simulink model "RoboBoat_CompassGPSlidar"  (R2014a)
settings: Solver=FixedStepDiscrete  StartTime=0.0  StopTime=inf  FixedStep=.1  RelTol=1e-3
undefined symbols (not defined in the file): Com1, Com2, Com3, Com4, DiscIntNeverNeededParam, standard
libraries: xpcseriallib x31, visiontextngfix x25, simulink x19, slrtlib x9, speedgoatlib_IO102 x3, speedgoatlib x2
(part 1 of 4)
settings Model: BufferReuse=off  Creator=wildcat  LastModifiedBy=wildcat
settings SolverCC: EnableConcurrentExecution=on
settings DataIOCC: SignalLoggingSaveFormat=ModelDataLogs
settings OptimizationCC: BlockReduction=off  OptimizeBlockIOStorage=off  BufferReuse=off  GlobalBufferReuse=off  ExpressionFolding=off  LocalBlockOutputs=off
settings DebuggingCC: UnderspecifiedInitializationDetection=Classic  MultiTaskDSMMsg=warning  StateNameClashWarn=warning
settings HardwareCC: ProdIntDivRoundTo=Zero  ProdEndianess=LittleEndian  ProdHWDeviceType=Generic->32-bit x86 compatible
settings RTWCC: SystemTargetFile=slrt.tlc  TemplateMakefile=slrt_default_tmf  Description=Simulink Real-Time  ProcessScript=slrt_make_rtw_hook  RTWCompilerOptimization=On
settings SimulinkRealTimeCC: GeneratePreprocessorConditionals=Disable all  EnableShiftOperators=on

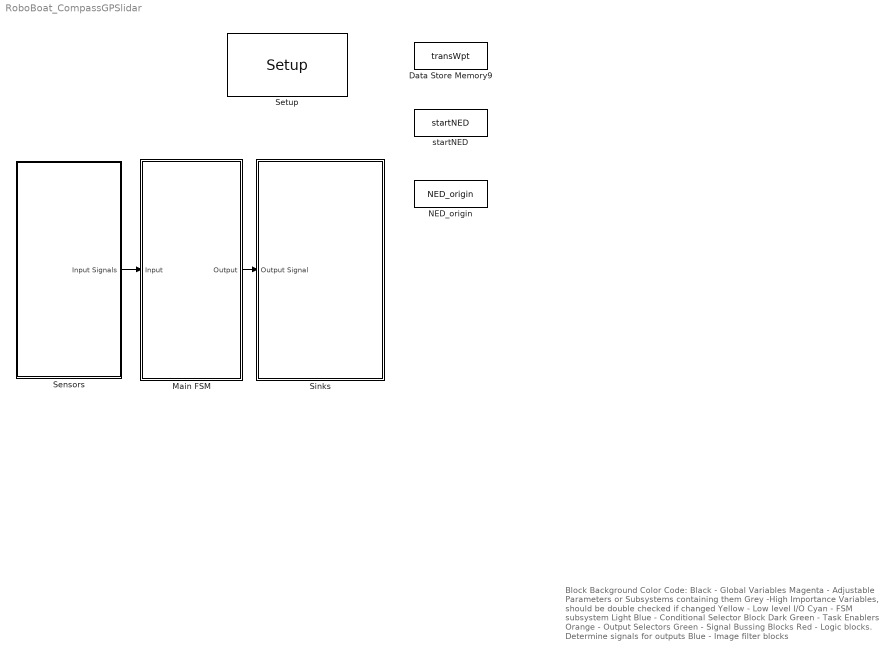
== system RoboBoat_CompassGPSlidar ==
  note: Block Background Color Code:
      | Black - Global Variables
      | Magenta - Adjustable Parameters or Subsystems containing them
      | Grey -High Importance Variables, should be double checked if changed
      | Yellow - Low level I/O
      | Cyan - FSM subsystem
      | Light Blue - Conditional Selector Block
      | Dark Green - Task Enablers
      | Orange - Output Selectors
      | Green - Signal Bussing Blocks
      | Red - Logic blocks. Determine signals for outputs
      | Blue - Image filter blocks
  Data Store Memory9 : DataStoreMemory  DataStoreName=transWpt  ReadBeforeWriteMsg=warning  WriteAfterWriteMsg=warning  WriteAfterReadMsg=warning  InitialValue=[4009.4964500000, 7532.95009000000]
  Main FSM : Subsystem
  NED_origin : DataStoreMemory  DataStoreName=NED_origin  ReadBeforeWriteMsg=warning  WriteAfterWriteMsg=warning  WriteAfterReadMsg=warning  InitialValue=[40.0395828333333, -74.6736588333333]  VectorParams1D=off
  Sensors : Subsystem
  Setup : speedgoatlib_IO102/Setup  group=Digital output setup  id=1  range=+-5V  cal=off  pciSlot=-1  adChannelMode=Multiple-channel (enter number of channels below)  adChannel=16  adCoupling=Differential  daChannel=[1,2,3,4]  daReset=[1]  daInitValue=[0]  diChannel=[1,2,3,4,5,6,7,8]  doChannel=[1,2,3,4,5,6,7,8]  doReset=[1]  doInitValue=[0]
  Sinks : Subsystem
  startNED : DataStoreMemory  DataStoreName=startNED  ReadBeforeWriteMsg=warning  WriteAfterWriteMsg=warning  WriteAfterReadMsg=warning  InitialValue=[10 10]  VectorParams1D=off
  wires:
  Sensors/1(Input Signals) -> Main FSM/1(Input)
  Main FSM/1(Output) -> Sinks/1(Output Signal)

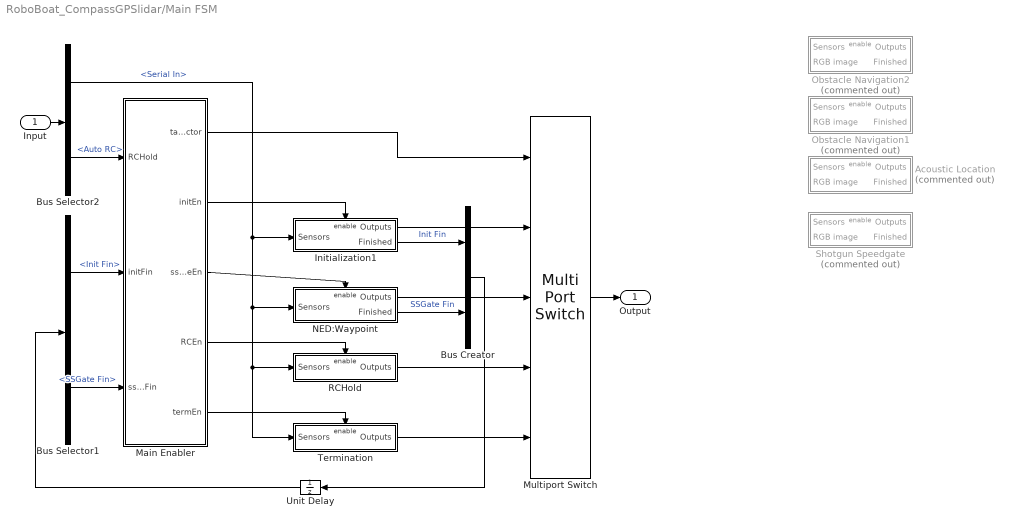
== system RoboBoat_CompassGPSlidar/Main FSM ==
  Input : Inport
  Acoustic Location : Subsystem  Commented=on  TreatAsAtomicUnit=on
  Bus Creator : BusCreator  Inputs=2
  Bus Selector1 : BusSelector  OutputSignals=Init Fin,SSGate Fin
  Bus Selector2 : BusSelector  OutputSignals=Serial In,Digital In.Auto RC
  Initialization1 : Subsystem
  Main Enabler : MATLAB Function  TreatAsAtomicUnit=on
  Multiport Switch : MultiPortSwitch  Inputs=4
  NED:Waypoint : Subsystem  TreatAsAtomicUnit=on
  Obstacle Navigation1 : Subsystem  Commented=on  TreatAsAtomicUnit=on
  Obstacle Navigation2 : Subsystem  Commented=on  TreatAsAtomicUnit=on
  RCHold : Subsystem
  Shotgun Speedgate : Subsystem  Commented=on  TreatAsAtomicUnit=on
  Termination : Subsystem  TreatAsAtomicUnit=on
  Unit Delay : UnitDelay  SampleTime=-1
  Output : Outport
  wires:
  Bus Creator/1 -> Unit Delay/1
  Initialization1/1(Outputs) -> Multiport Switch/2
  Multiport Switch/1 -> Output/1
  Main Enabler/1(taskSelector) -> Multiport Switch/1
  Initialization1/2(Finished) -> Bus Creator/1  "Init Fin"
  Unit Delay/1 -> Bus Selector1/1
  Input/1 -> Bus Selector2/1
  Main Enabler/2(initEn) -> Initialization1/Enable
  Termination/1(Outputs) -> Multiport Switch/5
  RCHold/1(Outputs) -> Multiport Switch/4
  Main Enabler/4(RCEn) -> RCHold/Enable
  Main Enabler/5(termEn) -> Termination/Enable
  Bus Selector2/1 -> Termination/1(Sensors), RCHold/1(Sensors), NED:Waypoint/1(Sensors), Initialization1/1(Sensors)  "<Serial In>"
  NED:Waypoint/2(Finished) -> Bus Creator/2  "SSGate Fin"
  NED:Waypoint/1(Outputs) -> Multiport Switch/3
  Main Enabler/3(ssGateEn) -> NED:Waypoint/Enable
  Bus Selector1/1 -> Main Enabler/2(initFin)  "<Init Fin>"
  Bus Selector1/2 -> Main Enabler/3(ssGateFin)  "<SSGate Fin>"
  Bus Selector2/2 -> Main Enabler/1(RCHold)  "<Auto RC>"

== system RoboBoat_CompassGPSlidar/Sensors ==
  1020 Comms : Subsystem  Commented=on
  Baseboard Serial : Subsystem
  Bus Creator : BusCreator  Inputs=2
  Digital In : Subsystem
  data log : Subsystem
  Input Signals : Outport
  wires:
  Baseboard Serial/1(Serial Inputs) -> Bus Creator/1
  Digital In/1(Digital In) -> Bus Creator/2
  Bus Creator/1 -> data log/1(Sensors signal), Input Signals/1  "Serial In"

== system RoboBoat_CompassGPSlidar/Sinks ==
  Output Signal : Inport
  Bus Selector : BusSelector  OutputSignals=Sensors.Compass.Heading,Outputs.Control Signals
  actuators : Subsystem
  wires:
  Bus Selector/2 -> actuators/2(Control Signals)  "<Control Signals>"
  Bus Selector/1 -> actuators/1(Compass Heading)  "<Heading>"
  Output Signal/1 -> Bus Selector/1

== system RoboBoat_CompassGPSlidar/Main FSM/Acoustic Location ==
  note: Acoustic Location
  Sensors : Inport
  RGB image : Inport  Port=2
  Enable : EnablePort  ShowOutputPort=on
  Annotate Task : visiontextngfix/Insert Text  inputType=Obsolete  theText='Acoustic Location...'  getTextLocFrom=Specify via dialog  textLoc=[10 10]  getTextColorFrom=Specify via dialog  textColor=[0 0 255]  getTextIntensityFrom=Specify via dialog  textIntensity=0  getTextOpacityFrom=Specify via dialog  textOpacity=1.0  dummyVar2=0  dummyVar3=0  dummyVar4=0  imagePorts=One multidimensional signal  isInputTransposed=off  fontFace=LucidaSansRegular  dummyVar1=0  blockFontSize=12  antiAliased=on
  Bus Selector : BusSelector  OutputSignals=Serial In.Compass.Heading
  Compare To Constant : simulink/Logic and Bit Operations/Compare To Constant  relop=>=  const=10  OutDataTypeStr=boolean
  Constant : Constant  Value=0
  Data Type Conversion : DataTypeConversion  OutDataTypeStr=double
  Discrete-Time Integrator : DiscreteIntegrator  SampleTime=0.1  ICPrevOutput=DiscIntNeverNeededParam  ICPrevScaledInput=DiscIntNeverNeededParam
  Output Heirarchy : Subsystem
  Outputs : Outport
  Finished : Outport  Port=2
  wires:
  Sensors/1 -> Output Heirarchy/3(Sensors), Bus Selector/1  "Sensors"
  Bus Selector/1 -> Output Heirarchy/2(Desired Heading)  "<Heading>"
  RGB image/1 -> Annotate Task/1
  Annotate Task/1 -> Output Heirarchy/1(Annotated Image)
  Output Heirarchy/1(Outputs) -> Outputs/1
  Compare To Constant/1 -> Data Type Conversion/1
  Enable/1 -> Discrete-Time Integrator/1
  Discrete-Time Integrator/1 -> Compare To Constant/1
  Constant/1 -> Output Heirarchy/4(Request Number)
  Data Type Conversion/1 -> Finished/1

== system RoboBoat_CompassGPSlidar/Main FSM/Initialization1 ==
  Sensors : Inport
  Enable : EnablePort  ShowOutputPort=on
  Bus Selector : BusSelector  OutputSignals=Compass.Heading
  Compare To Constant : simulink/Logic and Bit Operations/Compare To Constant  relop=>=  const=5  OutDataTypeStr=boolean
  Constant : Constant  Value=0
  Data Type Conversion : DataTypeConversion  OutDataTypeStr=double
  Discrete-Time Integrator : DiscreteIntegrator  SampleTime=-1  ICPrevOutput=DiscIntNeverNeededParam  ICPrevScaledInput=DiscIntNeverNeededParam
  Output Heirarchy : Subsystem
  Outputs : Outport
  Finished : Outport  Port=2
  wires:
  Sensors/1 -> Bus Selector/1, Output Heirarchy/2(Sensors)  "Sensors"
  Bus Selector/1 -> Output Heirarchy/1(Desired Heading)  "<Heading>"
  Output Heirarchy/1(Outputs) -> Outputs/1
  Compare To Constant/1 -> Data Type Conversion/1
  Enable/1 -> Discrete-Time Integrator/1
  Discrete-Time Integrator/1 -> Compare To Constant/1
  Constant/1 -> Output Heirarchy/3(Request Number)
  Data Type Conversion/1 -> Finished/1

== system RoboBoat_CompassGPSlidar/Main FSM/NED:Waypoint ==
  Sensors : Inport
  Enable : EnablePort
  Bus Selector2 : BusSelector  OutputSignals=GPS.X,GPS.Y,Compass.Heading
  Data Store Read3 : DataStoreRead  DataStoreName=startNED
  Demux : Demux  Outputs=2
  Model : ModelReference  ModelNameDialog=NEDnavV5.slx  SimulationMode=Normal  ModelReferenceVersion=1.2059  CopyOfModelName=NEDnavV5.slx  DefaultDataLogging=on
  Output Heirarchy : Subsystem
  Outputs : Outport
  Finished : Outport  Port=2
  wires:
  Model/1 -> Output Heirarchy/2(RPM)
  Model/2 -> Output Heirarchy/3(Desired Heading)
  Model/3 -> Finished/1
  Output Heirarchy/1(Outputs) -> Outputs/1
  Sensors/1 -> Bus Selector2/1, Output Heirarchy/1(Sensors)
  Bus Selector2/1 -> Model/1  "<X>"
  Bus Selector2/2 -> Model/2  "<Y>"
  Bus Selector2/3 -> Model/3  "<Heading>"
  Data Store Read3/1 -> Demux/1
  Demux/1 -> Model/4
  Demux/2 -> Model/5

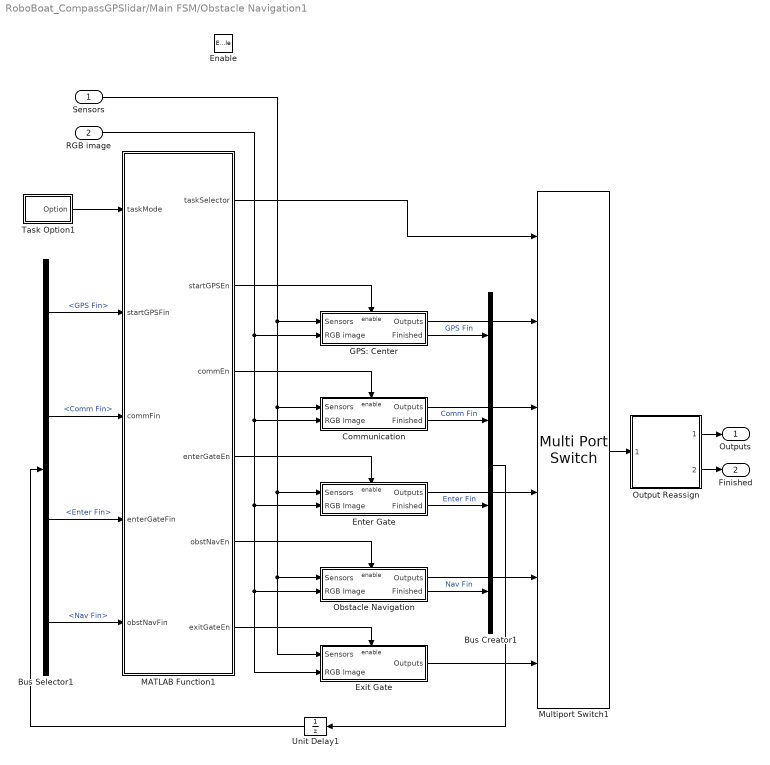
== system RoboBoat_CompassGPSlidar/Main FSM/Obstacle Navigation1 ==
  Sensors : Inport
  RGB image : Inport  Port=2
  Enable : EnablePort
  Bus Creator1 : BusCreator
  Bus Selector1 : BusSelector  OutputSignals=GPS Fin,Comm Fin,Enter Fin,Nav Fin
  Communication : Subsystem  TreatAsAtomicUnit=on
  Enter Gate : Subsystem  TreatAsAtomicUnit=on
  Exit Gate : Subsystem  TreatAsAtomicUnit=on
  GPS: Center : Subsystem  TreatAsAtomicUnit=on
  MATLAB Function1 : MATLAB Function  TreatAsAtomicUnit=on
  Multiport Switch1 : MultiPortSwitch  Inputs=5
  Obstacle Navigation : Subsystem  TreatAsAtomicUnit=on
  Output Reassign : Subsystem
  Task Option1 : Subsystem
  Unit Delay1 : UnitDelay  SampleTime=-1
  Outputs : Outport
  Finished : Outport  Port=2
  wires:
  Task Option1/1(Option) -> MATLAB Function1/1(taskMode)
  MATLAB Function1/2(startGPSEn) -> GPS: Center/Enable
  GPS: Center/1(Outputs) -> Multiport Switch1/2
  MATLAB Function1/1(taskSelector) -> Multiport Switch1/1
  MATLAB Function1/3(commEn) -> Communication/Enable
  MATLAB Function1/6(exitGateEn) -> Exit Gate/Enable
  MATLAB Function1/5(obstNavEn) -> Obstacle Navigation/Enable
  MATLAB Function1/4(enterGateEn) -> Enter Gate/Enable
  GPS: Center/2(Finished) -> Bus Creator1/1  "GPS Fin"
  Communication/2(Finished) -> Bus Creator1/2  "Comm Fin"
  Enter Gate/2(Finished) -> Bus Creator1/3  "Enter Fin"
  Obstacle Navigation/2(Finished) -> Bus Creator1/4  "Nav Fin"
  Obstacle Navigation/1(Outputs) -> Multiport Switch1/5
  Enter Gate/1(Outputs) -> Multiport Switch1/4
  Communication/1(Outputs) -> Multiport Switch1/3
  Bus Creator1/1 -> Unit Delay1/1
  Unit Delay1/1 -> Bus Selector1/1
  Bus Selector1/1 -> MATLAB Function1/2(startGPSFin)  "<GPS Fin>"
  Bus Selector1/2 -> MATLAB Function1/3(commFin)  "<Comm Fin>"
  Bus Selector1/3 -> MATLAB Function1/4(enterGateFin)  "<Enter Fin>"
  Bus Selector1/4 -> MATLAB Function1/5(obstNavFin)  "<Nav Fin>"
  Exit Gate/1(Outputs) -> Multiport Switch1/6
  Sensors/1 -> GPS: Center/1(Sensors), Communication/1(Sensors), Enter Gate/1(Sensors), Exit Gate/1(Sensors), Obstacle Navigation/1(Sensors)
  RGB image/1 -> GPS: Center/2(RGB image), Communication/2(RGB Image), Enter Gate/2(RGB Image), Exit Gate/2(RGB Image), Obstacle Navigation/2(RGB Image)
  Multiport Switch1/1 -> Output Reassign/1(Outputs in)
  Output Reassign/1(Outputs) -> Outputs/1
  Output Reassign/2(Finished) -> Finished/1

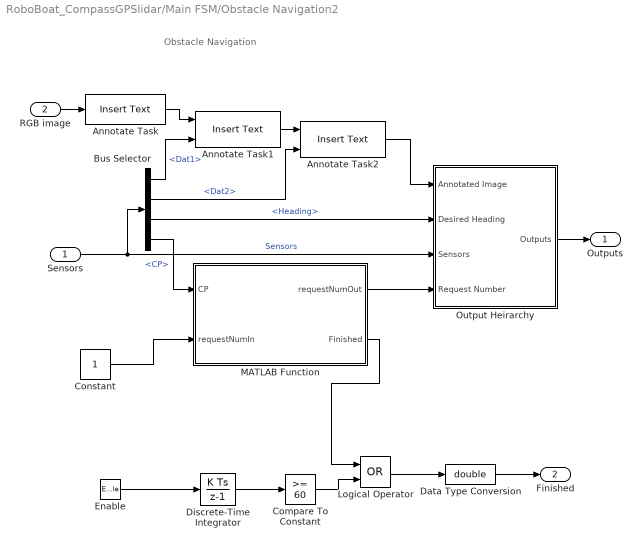
== system RoboBoat_CompassGPSlidar/Main FSM/Obstacle Navigation2 ==
  note: Obstacle Navigation
  Sensors : Inport
  RGB image : Inport  Port=2
  Enable : EnablePort  ShowOutputPort=on
  Annotate Task : visiontextngfix/Insert Text  inputType=Obsolete  theText='Obstacle Nav...'  getTextLocFrom=Specify via dialog  textLoc=[10 10]  getTextColorFrom=Specify via dialog  textColor=[0 0 255]  getTextIntensityFrom=Specify via dialog  textIntensity=0  getTextOpacityFrom=Specify via dialog  textOpacity=1.0  dummyVar2=0  dummyVar3=0  dummyVar4=0  imagePorts=One multidimensional signal  isInputTransposed=off  fontFace=LucidaSansRegular  dummyVar1=0  blockFontSize=12  antiAliased=on
  Annotate Task1 : visiontextngfix/Insert Text  inputType=Obsolete  theText='Enter Gate: %f'  getTextLocFrom=Specify via dialog  textLoc=[10 20]  getTextColorFrom=Specify via dialog  textColor=[0 0 255]  getTextIntensityFrom=Specify via dialog  textIntensity=0  getTextOpacityFrom=Specify via dialog  textOpacity=1.0  dummyVar2=0  dummyVar3=0  dummyVar4=0  imagePorts=One multidimensional signal  isInputTransposed=off  fontFace=LucidaSansRegular  dummyVar1=0  blockFontSize=12  antiAliased=on
  Annotate Task2 : visiontextngfix/Insert Text  inputType=Obsolete  theText='Exit Gate: %f'  getTextLocFrom=Specify via dialog  textLoc=[10 30]  getTextColorFrom=Specify via dialog  textColor=[0 0 255]  getTextIntensityFrom=Specify via dialog  textIntensity=0  getTextOpacityFrom=Specify via dialog  textOpacity=1.0  dummyVar2=0  dummyVar3=0  dummyVar4=0  imagePorts=One multidimensional signal  isInputTransposed=off  fontFace=LucidaSansRegular  dummyVar1=0  blockFontSize=12  antiAliased=on
  Bus Selector : BusSelector  OutputSignals=Serial In.Comms.Dat1,Serial In.Comms.Dat2,Serial In.Compass.Heading,Serial In.Comms.CP
  Compare To Constant : simulink/Logic and Bit Operations/Compare To Constant  relop=>=  const=60  OutDataTypeStr=boolean
  Constant : Constant
  Data Type Conversion : DataTypeConversion  OutDataTypeStr=double
  Discrete-Time Integrator : DiscreteIntegrator  SampleTime=0.1  ICPrevOutput=DiscIntNeverNeededParam  ICPrevScaledInput=DiscIntNeverNeededParam
  Logical Operator : Logic  Operator=OR  AllPortsSameDT=off  OutDataTypeStr=boolean
  MATLAB Function : MATLAB Function  TreatAsAtomicUnit=on
  Output Heirarchy : Subsystem
  Outputs : Outport
  Finished : Outport  Port=2
  wires:
  Sensors/1 -> Bus Selector/1, Output Heirarchy/3(Sensors)  "Sensors"
  Bus Selector/3 -> Output Heirarchy/2(Desired Heading)  "<Heading>"
  RGB image/1 -> Annotate Task/1
  Output Heirarchy/1(Outputs) -> Outputs/1
  Enable/1 -> Discrete-Time Integrator/1
  Discrete-Time Integrator/1 -> Compare To Constant/1
  Annotate Task/1 -> Annotate Task1/1
  Bus Selector/1 -> Annotate Task1/2  "<Dat1>"
  Annotate Task1/1 -> Annotate Task2/1
  Bus Selector/2 -> Annotate Task2/2  "<Dat2>"
  Annotate Task2/1 -> Output Heirarchy/1(Annotated Image)
  Data Type Conversion/1 -> Finished/1
  MATLAB Function/2(Finished) -> Logical Operator/1
  Compare To Constant/1 -> Logical Operator/2
  Logical Operator/1 -> Data Type Conversion/1
  MATLAB Function/1(requestNumOut) -> Output Heirarchy/4(Request Number)
  Constant/1 -> MATLAB Function/2(requestNumIn)
  Bus Selector/4 -> MATLAB Function/1(CP)  "<CP>"

== system RoboBoat_CompassGPSlidar/Main FSM/RCHold ==
  Sensors : Inport
  Enable : EnablePort
  Bus Selector : BusSelector  OutputSignals=Compass.Heading
  Output Heirarchy : Subsystem
  Outputs : Outport
  wires:
  Sensors/1 -> Output Heirarchy/2(Sensors), Bus Selector/1  "Sensors"
  Bus Selector/1 -> Output Heirarchy/1(Desired Heading)  "<Heading>"
  Output Heirarchy/1(Outputs) -> Outputs/1

== system RoboBoat_CompassGPSlidar/Main FSM/Shotgun Speedgate ==
  note: Start Speed Gate
  Sensors : Inport
  RGB image : Inport  Port=2
  Enable : EnablePort  ShowOutputPort=on
  Bus Selector : BusSelector  OutputSignals=Serial In.Compass.Heading
  Compare To Constant : simulink/Logic and Bit Operations/Compare To Constant  relop=>=  const=60  OutDataTypeStr=boolean
  Constant : Constant  Value=4000
  Data Type Conversion : DataTypeConversion  OutDataTypeStr=double
  Insert Text : visiontextngfix/Insert Text  inputType=Obsolete  theText='SSGate Shotgun'  getTextLocFrom=Specify via dialog  textLoc=[1 1]  getTextColorFrom=Specify via dialog  textColor=[0 0 0]  getTextIntensityFrom=Specify via dialog  textIntensity=0  getTextOpacityFrom=Specify via dialog  textOpacity=1.0  dummyVar2=0  dummyVar3=0  dummyVar4=0  imagePorts=One multidimensional signal  isInputTransposed=off  fontFace=LucidaSansRegular  dummyVar1=0  blockFontSize=12  antiAliased=on
  MATLAB Function : MATLAB Function  TreatAsAtomicUnit=on
  MATLAB Function1 : MATLAB Function  TreatAsAtomicUnit=on
  Output Heirarchy : Subsystem
  "Scope " : slrtlib/Displays and Logging/Scope   scopeno=1  scopetype=File  autostart=on  viewmode=Graphical redraw  formatstr='%15.6f'  grid=on  ylimits=[0,0]  nosamples=300  noprepostsamples=0  interleave=1  triggermode=FreeRun  triggersignal=1  trigsignalfromport=off  triggerlevel=0.0  triggerslope=Either  triggerscope=1  triggersample=0  filename=ssgate.dat  mode=Lazy  writesize=512  autorestart=off  dynamicfilemode=off  maxwritefilesize=512*1024^2
  Timer : DiscreteIntegrator  SampleTime=-1  ICPrevOutput=DiscIntNeverNeededParam  ICPrevScaledInput=DiscIntNeverNeededParam
  Outputs : Outport
  Finished : Outport  Port=2
  wires:
  RGB image/1 -> Insert Text/1
  Sensors/1 -> Output Heirarchy/1(Sensors), Bus Selector/1  "Sensors"
  Enable/1 -> Timer/1
  Timer/1 -> Compare To Constant/1
  Output Heirarchy/1(Outputs) -> Outputs/1
  Data Type Conversion/1 -> Finished/1
  Compare To Constant/1 -> Data Type Conversion/1
  Constant/1 -> Output Heirarchy/3(RPM)
  Bus Selector/1 -> MATLAB Function1/2(Heading), MATLAB Function/1(Heading)  "<Heading>"
  MATLAB Function/1(LockedHeading) -> MATLAB Function1/1(desiredHeading), Output Heirarchy/4(Desired Heading)
  Insert Text/1 -> Output Heirarchy/2(Annotated Image)
  MATLAB Function1/1(out) -> "Scope "/1

== system RoboBoat_CompassGPSlidar/Main FSM/Termination ==
  Sensors : Inport
  Enable : EnablePort
  Bus Selector : BusSelector  OutputSignals=Compass.Heading
  Output Heirarchy : Subsystem
  Outputs : Outport
  wires:
  Output Heirarchy/1(Outputs) -> Outputs/1
  Sensors/1 -> Bus Selector/1, Output Heirarchy/2(Sensors)  "Sensors"
  Bus Selector/1 -> Output Heirarchy/1(Desired Heading)  "<Heading>"

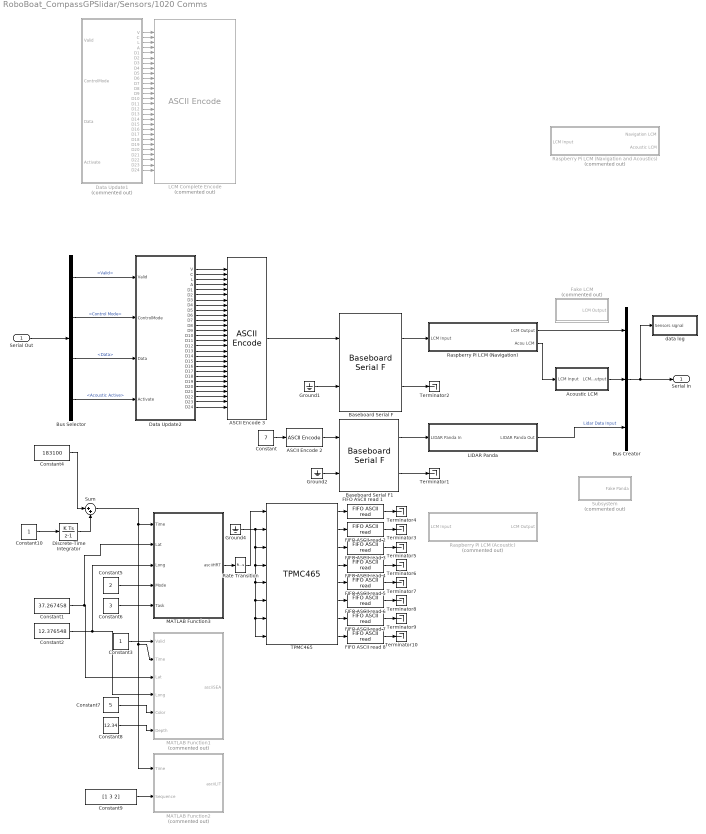
== system RoboBoat_CompassGPSlidar/Sensors/1020 Comms ==
  Serial Out : Inport
  " Raspberry Pi LCM (Acoustic)" : Subsystem  Commented=on
  " Raspberry Pi LCM (Navigation and Acoustics)" : Subsystem  Commented=on
  " Raspberry Pi LCM (Navigation)" : Subsystem
  ASCII Encode 2 : xpcseriallib/ASCII Encode   format=SGTask:%d \r\n  nvars=1  maxlength=128  vartypes={ 'double' }
  ASCII Encode 3 : xpcseriallib/ASCII Encode   format="{\"Valid\":%d, \"Mode\":%d, \"Length\":%d, \"Activate\":%d, \"Waypoints\":[%f, %f, %f, %f, %f, %f, %f, %f, %f, %f, %f, %f, %f, %f, %f, %f, %f, %f, %f, %f, %f, %f, %f, %f]} \\r\\n"  nvars=28  maxlength=1000  vartypes={ 'double' }
  Acoustic LCM : Subsystem
  Baseboard Serial F : xpcseriallib/Mainboard/Baseboard Serial F  group=Basic Setup  port=1  irqnum=4  saddr1=0x3f8  saddr2=0x3e8  config=Com1/Com3  baud1=115200  parity1=Even  ndata1=7  nstop1=1  fifomode1=64 deep  rlevel1=1  automode1=on  xmtfifosize1=1024  xmtdatatype1=8 bit uint null terminated  rcvfifosize1=1024  baud2=115200  parity2=Even  ndata2=7  nstop2=1  fifomode2=64 deep  rlevel2=1  automode2=on  xmtfifosize2=1024  xmtdatatype2=8 bit uint null terminated  rcvfifosize2=1024
  Baseboard Serial F1 : xpcseriallib/Mainboard/Baseboard Serial F  group=FIFO Setup  port=1  irqnum=4  saddr1=0x3f8  saddr2=0x3e8  config=Com2/Com4  baud1=115200  parity1=Even  ndata1=7  nstop1=1  fifomode1=64 deep  rlevel1=1  automode1=on  xmtfifosize1=1024  xmtdatatype1=8 bit uint null terminated  rcvfifosize1=1024  baud2=115200  parity2=Even  ndata2=7  nstop2=1  fifomode2=64 deep  rlevel2=1  automode2=on  xmtfifosize2=1024  xmtdatatype2=8 bit uint null terminated  rcvfifosize2=1024
  Bus Creator : BusCreator  Inputs=3
  Bus Selector : BusSelector  OutputSignals=Outputs.Navigation Outputs.Valid,Outputs.Navigation Outputs.Control Mode,Outputs.Navigation Outputs.Data,Outputs.Acoustic Active
  Constant : Constant  Value=7
  Constant1 : Constant  Value=37.267458
  Constant10 : Constant
  Constant2 : Constant  Value=12.376548
  Constant3 : Constant
  Constant4 : Constant  Value=183100
  Constant5 : Constant  Value=2
  Constant6 : Constant  Value=3
  Constant7 : Constant  Value=5
  Constant8 : Constant  Value=12.34
  Constant9 : Constant  Value=[1 3 2]
  Data Update1 : MATLAB Function  Commented=on  TreatAsAtomicUnit=on
  Data Update2 : MATLAB Function  TreatAsAtomicUnit=on
  Discrete-Time Integrator : DiscreteIntegrator  SampleTime=-1  ICPrevOutput=DiscIntNeverNeededParam  ICPrevScaledInput=DiscIntNeverNeededParam
  FIFO ASCII read {1..8} (8 alike) : xpcseriallib/FIFO ASCII read   header={'Deploy:'}  term=[13 10]  hold=Zero output if no new data  enable=off  maxsize=1024  outputtype=8 bit uint null terminated  sampletime=-1
  Fake LCM : Subsystem  Commented=on
  Ground1 : Ground
  Ground2 : Ground
  Ground4 : Ground
  LCM Complete Encode : xpcseriallib/ASCII Encode   Commented=on  format="{\"Valid\":%d, \"Mode\":%d, \"Length\":%d, \"Activate\":%d, \"Waypoints\":[%f, %f, %f, %f, %f, %f, %f, %f, %f, %f, %f, %f, %f, %f, %f, %f, %f, %f, %f, %f, %f, %f, %f, %f]} \\r\\n"  nvars=28  maxlength=1000  vartypes={ 'double' }
  LIDAR Panda : Subsystem
  MATLAB Function1 : MATLAB Function  Commented=on  TreatAsAtomicUnit=on
  MATLAB Function2 : MATLAB Function  Commented=on  TreatAsAtomicUnit=on
  MATLAB Function3 : MATLAB Function  TreatAsAtomicUnit=on
  Rate Transition : RateTransition  Deterministic=off  OutPortSampleTime=1
  Subsystem : Subsystem  Commented=on
  Sum : Sum  Inputs=|++
  TPMC465 : speedgoatlib/IO504/TPMC465  group=Basic Setup  port=2  irqnum=9  slot=-1  transceiver1=RS232 (max 921.6kb/s)  standard1=on  baud1=115200  bauddivisor1=1  sampling1=16x (standard)  prescale1=off  parity1=Even  ndata1=7  nstop1=1  rlevel1=half full (32)  hwmode1=none  swmode1=none  xonchar1=17  xoffchar1=19  rs485auto1=off  rs485delay1=0  xmtfifosize1=1024  xmtdatatype1=8 bit uint null terminated  rcvfifosize1=1024  transceiver2=RS232 (max 921.6kb/s)  standard2=on  baud2=115200  bauddivisor2=1  sampling2=16x (standard)  prescale2=off  parity2=Even  ndata2=7  nstop2=1  rlevel2=half full (32)  hwmode2=none  swmode2=none  xonchar2=17  xoffchar2=19  rs485auto2=off  rs485delay2=0  xmtfifosize2=1024  xmtdatatype2=8 bit uint null terminated  rcvfifosize2=1024  transceiver3=RS232 (max 921.6kb/s)  standard3=on  baud3=115200  bauddivisor3=1  sampling3=16x (standard)  prescale3=off  parity3=Even  ndata3=7  nstop3=1  rlevel3=half full (32)  hwmode3=none  swmode3=none  xonchar3=17  xoffchar3=19  rs485auto3=off  rs485delay3=0  xmtfifosize3=1024  xmtdatatype3=8 bit uint null terminated  rcvfifosize3=1024  transceiver4=RS232 (max 921.6kb/s)  standard4=on  baud4=115200  bauddivisor4=1  sampling4=16x (standard)  prescale4=off  parity4=None  ndata4=8  nstop4=1  rlevel4=half full (32)  hwmode4=none  swmode4=none  xonchar4=17  xoffchar4=19  rs485auto4=off  rs485delay4=0  xmtfifosize4=1024  xmtdatatype4=8 bit uint null terminated  rcvfifosize4=1024  transceiver5=RS232 (max 921.6kb/s)  standard5=on  baud5=115200  bauddivisor5=1  sampling5=16x (standard)  prescale5=off  parity5=None  ndata5=8  nstop5=1  rlevel5=1  hwmode5=none  swmode5=none  xonchar5=17  xoffchar5=19  rs485auto5=off  rs485delay5=0  xmtfifosize5=1024  xmtdatatype5=8 bit uint null terminated  rcvfifosize5=1024  transceiver6=RS232 (max 921.6kb/s)  standard6=on  baud6=115200  bauddivisor6=1  sampling6=16x (standard)  prescale6=off  parity6=None  ndata6=8  nstop6=1  rlevel6=1  hwmode6=none  swmode6=none  xonchar6=17  xoffchar6=19  rs485auto6=off  rs485delay6=0  xmtfifosize6=1024  xmtdatatype6=8 bit uint null terminated  rcvfifosize6=1024  transceiver7=RS232 (max 921.6kb/s)  standard7=on  baud7=115200  bauddivisor7=1  sampling7=16x (standard)  prescale7=off  parity7=None  ndata7=8  nstop7=1  rlevel7=1  hwmode7=none  swmode7=none  xonchar7=17  xoffchar7=19  rs485auto7=off  rs485delay7=0  xmtfifosize7=1024  xmtdatatype7=8 bit uint null terminated  rcvfifosize7=1024  transceiver8=RS232 (max 921.6kb/s)  standard8=on  baud8=115200  bauddivisor8=1  sampling8=16x (standard)  prescale8=off  parity8=None  ndata8=8  nstop8=1  rlevel8=1  hwmode8=none  swmode8=none  xonchar8=17  xoffchar8=19  rs485auto8=off  rs485delay8=0  xmtfifosize8=1024  xmtdatatype8=8 bit uint null terminated  rcvfifosize8=1024
  Terminator{1..10} (10 alike) : Terminator
  data log : Subsystem
  Serial In : Outport
  wires:
  Serial Out/1 -> Bus Selector/1
  Baseboard Serial F/1 -> " Raspberry Pi LCM (Navigation)"/1(LCM Input)
  ASCII Encode 3/1 -> Baseboard Serial F/1
  " Raspberry Pi LCM (Navigation)"/1(LCM Output) -> Bus Creator/1
  Bus Selector/1 -> Data Update2/1(Valid)  "<Valid>"
  Bus Selector/2 -> Data Update2/2(ControlMode)  "<Control Mode>"
  Bus Selector/3 -> Data Update2/3(Data)  "<Data>"
  Acoustic LCM/1(LCM Output) -> Bus Creator/2
  Baseboard Serial F/2 -> Terminator2/1
  Ground1/1 -> Baseboard Serial F/2
  LIDAR Panda/1(LIDAR Panda Out) -> Bus Creator/3  "Lidar Data Input"
  Bus Creator/1 -> Serial In/1, data log/1(Sensors signal)
  Data Update1/1(V) -> LCM Complete Encode/1
  Data Update1/2(C) -> LCM Complete Encode/2
  Data Update1/6(D2) -> LCM Complete Encode/6
  Data Update1/7(D3) -> LCM Complete Encode/7
  Data Update1/8(D4) -> LCM Complete Encode/8
  Data Update1/5(D1) -> LCM Complete Encode/5
  Data Update1/9(D5) -> LCM Complete Encode/9
  Data Update1/10(D6) -> LCM Complete Encode/10
  Data Update1/11(D7) -> LCM Complete Encode/11
  Data Update1/12(D8) -> LCM Complete Encode/12
  Data Update1/13(D9) -> LCM Complete Encode/13
  Data Update1/18(D14) -> LCM Complete Encode/18
  Data Update1/15(D11) -> LCM Complete Encode/15
  Data Update1/20(D16) -> LCM Complete Encode/20
  Data Update1/21(D17) -> LCM Complete Encode/21
  Data Update1/19(D15) -> LCM Complete Encode/19
  Data Update1/14(D10) -> LCM Complete Encode/14
  Data Update1/16(D12) -> LCM Complete Encode/16
  Data Update1/22(D18) -> LCM Complete Encode/22
  Data Update1/23(D19) -> LCM Complete Encode/23
  Data Update1/24(D20) -> LCM Complete Encode/24
  Data Update1/25(D21) -> LCM Complete Encode/25
  Data Update1/27(D23) -> LCM Complete Encode/27
  Data Update1/26(D22) -> LCM Complete Encode/26
  Data Update1/28(D24) -> LCM Complete Encode/28
  Data Update1/3(L) -> LCM Complete Encode/3
  Data Update1/4(A) -> LCM Complete Encode/4
  Data Update1/17(D13) -> LCM Complete Encode/17
  " Raspberry Pi LCM (Navigation)"/2(Acou LCM) -> Acoustic LCM/1(LCM Input)
  Data Update2/21(D17) -> ASCII Encode 3/21
  Data Update2/20(D16) -> ASCII Encode 3/20
  Data Update2/19(D15) -> ASCII Encode 3/19
  Data Update2/4(A) -> ASCII Encode 3/4
  Data Update2/2(C) -> ASCII Encode 3/2
  Data Update2/18(D14) -> ASCII Encode 3/18
  Data Update2/16(D12) -> ASCII Encode 3/16
  Data Update2/7(D3) -> ASCII Encode 3/7
  Data Update2/6(D2) -> ASCII Encode 3/6
  Data Update2/5(D1) -> ASCII Encode 3/5
  Data Update2/17(D13) -> ASCII Encode 3/17
  Data Update2/9(D5) -> ASCII Encode 3/9
  Data Update2/10(D6) -> ASCII Encode 3/10
  Data Update2/24(D20) -> ASCII Encode 3/24
  Data Update2/23(D19) -> ASCII Encode 3/23
  Data Update2/28(D24) -> ASCII Encode 3/28
  Data Update2/26(D22) -> ASCII Encode 3/26
  Data Update2/25(D21) -> ASCII Encode 3/25
  Data Update2/3(L) -> ASCII Encode 3/3
  Data Update2/27(D23) -> ASCII Encode 3/27
  Data Update2/8(D4) -> ASCII Encode 3/8
  Data Update2/11(D7) -> ASCII Encode 3/11
  Data Update2/13(D9) -> ASCII Encode 3/13
  Data Update2/12(D8) -> ASCII Encode 3/12
  Data Update2/14(D10) -> ASCII Encode 3/14
  Data Update2/22(D18) -> ASCII Encode 3/22
  Data Update2/15(D11) -> ASCII Encode 3/15
  Bus Selector/4 -> Data Update2/4(Activate)  "<Acoustic Active>"
  Data Update2/1(V) -> ASCII Encode 3/1
  Constant9/1 -> MATLAB Function2/2(Sequence)
  Constant7/1 -> MATLAB Function1/5(Color)
  Constant8/1 -> MATLAB Function1/6(Depth)
  Constant5/1 -> MATLAB Function3/4(Mode)
  Constant6/1 -> MATLAB Function3/5(Task)
  Sum/1 -> MATLAB Function3/1(Time), MATLAB Function2/1(Time), MATLAB Function1/2(Time)
  Constant2/1 -> MATLAB Function3/3(Long), MATLAB Function1/4(Long)
  Constant1/1 -> MATLAB Function3/2(Lat), MATLAB Function1/3(Lat)
  Ground4/1 -> TPMC465/2, TPMC465/3, TPMC465/4, TPMC465/8, TPMC465/7, TPMC465/6, TPMC465/5
  TPMC465/1 -> FIFO ASCII read 1/1
  FIFO ASCII read 1/1 -> Terminator4/1
  FIFO ASCII read 2/1 -> Terminator3/1
  FIFO ASCII read 3/1 -> Terminator5/1
  FIFO ASCII read 4/1 -> Terminator6/1
  FIFO ASCII read 5/1 -> Terminator7/1
  FIFO ASCII read 6/1 -> Terminator8/1
  FIFO ASCII read 7/1 -> Terminator9/1
  FIFO ASCII read 8/1 -> Terminator10/1
  TPMC465/2 -> FIFO ASCII read 2/1
  TPMC465/3 -> FIFO ASCII read 3/1
  TPMC465/4 -> FIFO ASCII read 4/1
  TPMC465/5 -> FIFO ASCII read 5/1
  TPMC465/6 -> FIFO ASCII read 6/1
  TPMC465/7 -> FIFO ASCII read 7/1
  TPMC465/8 -> FIFO ASCII read 8/1
  Rate Transition/1 -> TPMC465/1
  Constant3/1 -> MATLAB Function1/1(Valid)
  MATLAB Function3/1(asciiHRT) -> Rate Transition/1
  Constant4/1 -> Sum/1
  Discrete-Time Integrator/1 -> Sum/2
  Constant10/1 -> Discrete-Time Integrator/1
  Baseboard Serial F1/1 -> LIDAR Panda/1(LIDAR Panda In)
  Ground2/1 -> Baseboard Serial F1/2
  Baseboard Serial F1/2 -> Terminator1/1
  ASCII Encode 2/1 -> Baseboard Serial F1/1
  Constant/1 -> ASCII Encode 2/1

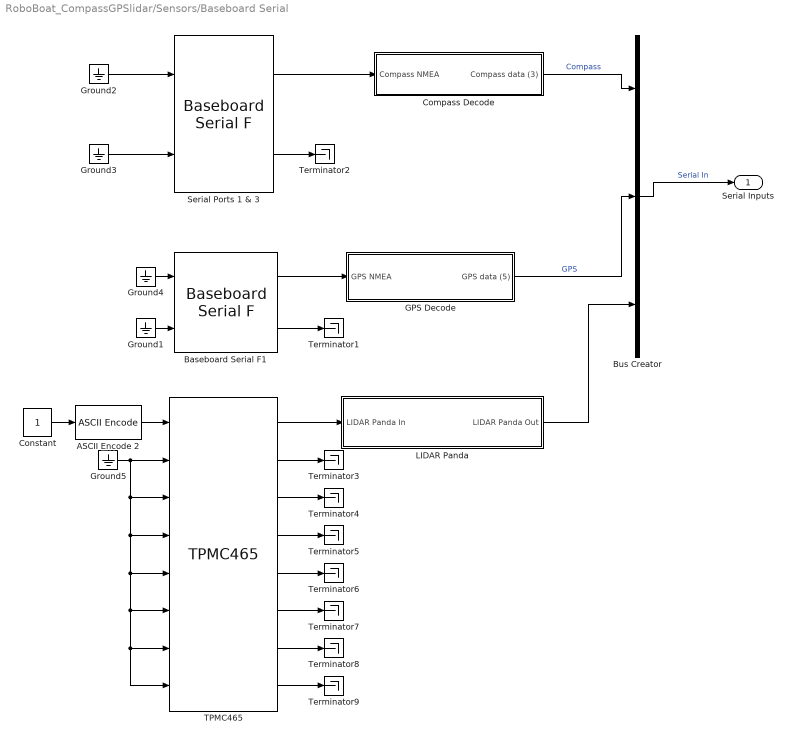
== system RoboBoat_CompassGPSlidar/Sensors/Baseboard Serial ==
  ASCII Encode 2 : xpcseriallib/ASCII Encode   format=SGTask:%d \r\n  nvars=1  maxlength=128  vartypes={ 'double' }
  Baseboard Serial F1 : xpcseriallib/Mainboard/Baseboard Serial F  group=Basic Setup  port=1  irqnum=4  saddr1=0x3f8  saddr2=0x3e8  config=Com2/Com4  baud1=19200  parity1=None  ndata1=8  nstop1=1  fifomode1=64 deep  rlevel1=half full  automode1=on  xmtfifosize1=1024  xmtdatatype1=8 bit uint null terminated  rcvfifosize1=1024  baud2=115200  parity2=Even  ndata2=7  nstop2=1  fifomode2=64 deep  rlevel2=1  automode2=on  xmtfifosize2=1024  xmtdatatype2=8 bit uint null terminated  rcvfifosize2=1024
  Bus Creator : BusCreator  Inputs=3
  Compass Decode : Subsystem
  Constant : Constant
  GPS Decode : Subsystem
  Ground{1..5} (5 alike) : Ground
  LIDAR Panda : Subsystem
  Serial Ports 1 & 3 : xpcseriallib/Mainboard/Baseboard Serial F  group=Basic Setup  port=2  irqnum=4  saddr1=0x3f8  saddr2=0x3e8  config=Com1/Com3  baud1=19200  parity1=None  ndata1=8  nstop1=1  fifomode1=64 deep  rlevel1=half full  automode1=off  xmtfifosize1=1024  xmtdatatype1=8 bit uint null terminated  rcvfifosize1=1024  baud2=19200  parity2=None  ndata2=8  nstop2=1  fifomode2=64 deep  rlevel2=half full  automode2=off  xmtfifosize2=1024  xmtdatatype2=8 bit uint null terminated  rcvfifosize2=1024
  TPMC465 : speedgoatlib/IO504/TPMC465  group=Basic Setup  port=1  irqnum=9  slot=-1  transceiver1=RS232 (max 921.6kb/s)  standard1=on  baud1=115200  bauddivisor1=1  sampling1=16x (standard)  prescale1=off  parity1=None  ndata1=8  nstop1=1  rlevel1=half full (32)  hwmode1=none  swmode1=none  xonchar1=17  xoffchar1=19  rs485auto1=off  rs485delay1=0  xmtfifosize1=1024  xmtdatatype1=8 bit uint null terminated  rcvfifosize1=1024  transceiver2=RS232 (max 921.6kb/s)  standard2=on  baud2=115200  bauddivisor2=1  sampling2=16x (standard)  prescale2=off  parity2=None  ndata2=8  nstop2=1  rlevel2=half full (32)  hwmode2=none  swmode2=none  xonchar2=17  xoffchar2=19  rs485auto2=off  rs485delay2=0  xmtfifosize2=1024  xmtdatatype2=8 bit uint null terminated  rcvfifosize2=1024  transceiver3=RS232 (max 921.6kb/s)  standard3=on  baud3=115200  bauddivisor3=1  sampling3=16x (standard)  prescale3=off  parity3=None  ndata3=8  nstop3=1  rlevel3=half full (32)  hwmode3=none  swmode3=none  xonchar3=17  xoffchar3=19  rs485auto3=off  rs485delay3=0  xmtfifosize3=1024  xmtdatatype3=8 bit uint null terminated  rcvfifosize3=1024  transceiver4=RS232 (max 921.6kb/s)  standard4=on  baud4=115200  bauddivisor4=1  sampling4=16x (standard)  prescale4=off  parity4=None  ndata4=8  nstop4=1  rlevel4=half full (32)  hwmode4=none  swmode4=none  xonchar4=17  xoffchar4=19  rs485auto4=off  rs485delay4=0  xmtfifosize4=1024  xmtdatatype4=8 bit uint null terminated  rcvfifosize4=1024  transceiver5=RS232 (max 921.6kb/s)  standard5=on  baud5=115200  bauddivisor5=1  sampling5=16x (standard)  prescale5=off  parity5=None  ndata5=8  nstop5=1  rlevel5=1  hwmode5=none  swmode5=none  xonchar5=17  xoffchar5=19  rs485auto5=off  rs485delay5=0  xmtfifosize5=1024  xmtdatatype5=8 bit uint null terminated  rcvfifosize5=1024  transceiver6=RS232 (max 921.6kb/s)  standard6=on  baud6=115200  bauddivisor6=1  sampling6=16x (standard)  prescale6=off  parity6=None  ndata6=8  nstop6=1  rlevel6=1  hwmode6=none  swmode6=none  xonchar6=17  xoffchar6=19  rs485auto6=off  rs485delay6=0  xmtfifosize6=1024  xmtdatatype6=8 bit uint null terminated  rcvfifosize6=1024  transceiver7=RS232 (max 921.6kb/s)  standard7=on  baud7=115200  bauddivisor7=1  sampling7=16x (standard)  prescale7=off  parity7=None  ndata7=8  nstop7=1  rlevel7=1  hwmode7=none  swmode7=none  xonchar7=17  xoffchar7=19  rs485auto7=off  rs485delay7=0  xmtfifosize7=1024  xmtdatatype7=8 bit uint null terminated  rcvfifosize7=1024  transceiver8=RS232 (max 921.6kb/s)  standard8=on  baud8=115200  bauddivisor8=1  sampling8=16x (standard)  prescale8=off  parity8=None  ndata8=8  nstop8=1  rlevel8=1  hwmode8=none  swmode8=none  xonchar8=17  xoffchar8=19  rs485auto8=off  rs485delay8=0  xmtfifosize8=1024  xmtdatatype8=8 bit uint null terminated  rcvfifosize8=1024
  Terminator{1..9} (9 alike) : Terminator
  Serial Inputs : Outport
  wires:
  Ground2/1 -> Serial Ports 1 & 3/1
  Ground3/1 -> Serial Ports 1 & 3/2
  Serial Ports 1 & 3/1 -> Compass Decode/1(Compass NMEA)
  GPS Decode/1(GPS data (5)) -> Bus Creator/2  "GPS"
  Compass Decode/1(Compass data (3)) -> Bus Creator/1  "Compass"
  Bus Creator/1 -> Serial Inputs/1  "Serial In"
  Baseboard Serial F1/1 -> GPS Decode/1(GPS NMEA)
  Ground1/1 -> Baseboard Serial F1/2
  Baseboard Serial F1/2 -> Terminator1/1
  Serial Ports 1 & 3/2 -> Terminator2/1
  Constant/1 -> ASCII Encode 2/1
  Ground4/1 -> Baseboard Serial F1/1
  ASCII Encode 2/1 -> TPMC465/1
  TPMC465/1 -> LIDAR Panda/1(LIDAR Panda In)
  TPMC465/2 -> Terminator3/1
  TPMC465/3 -> Terminator4/1
  TPMC465/4 -> Terminator5/1
  TPMC465/5 -> Terminator6/1
  TPMC465/6 -> Terminator7/1
  TPMC465/7 -> Terminator8/1
  TPMC465/8 -> Terminator9/1
  Ground5/1 -> TPMC465/3, TPMC465/4, TPMC465/5, TPMC465/6, TPMC465/7, TPMC465/8, TPMC465/2
  LIDAR Panda/1(LIDAR Panda Out) -> Bus Creator/3

== system RoboBoat_CompassGPSlidar/Sensors/Digital In ==
  Bus Creator : BusCreator  Inputs=1
  Digital input : speedgoatlib_IO102/Digital input  id=1  channels=[1,2,3,4,5,6,7,8]  ts=-1  pciSlot=-1
  Terminator{1,17..22} (7 alike) : Terminator
  Digital In : Outport
  wires:
  Bus Creator/1 -> Digital In/1  "Digital In"
  Digital input/8 -> Bus Creator/1  "Auto RC"
  Digital input/2 -> Terminator17/1
  Digital input/3 -> Terminator18/1
  Digital input/4 -> Terminator19/1
  Digital input/5 -> Terminator20/1
  Digital input/6 -> Terminator21/1
  Digital input/7 -> Terminator22/1
  Digital input/1 -> Terminator1/1

== system RoboBoat_CompassGPSlidar/Sensors/data log ==
  Sensors signal : Inport
  Bus to Vector : BusToVector
  Scope 2 : slrtlib/Displays and Logging/Scope   scopeno=1  scopetype=File  autostart=on  viewmode=Graphical redraw  formatstr='%15.6f'  grid=on  ylimits=[0,0]  nosamples=250  noprepostsamples=0  interleave=1  triggermode=FreeRun  triggersignal=1  trigsignalfromport=off  triggerlevel=0.0  triggerslope=Either  triggerscope=1  triggersample=0  filename=NW9_<%%%>.dat  mode=Commit  writesize=512  autorestart=on  dynamicfilemode=on  maxwritefilesize=512*1024^2
  wires:
  Sensors signal/1 -> Bus to Vector/1
  Bus to Vector/1 -> Scope 2/1

== system RoboBoat_CompassGPSlidar/Sinks/actuators ==
  Compass Heading : Inport
  Control Signals : Inport  Port=2
  analog output : Subsystem
  wires:
  Control Signals/1 -> analog output/2(Control Signals)
  Compass Heading/1 -> analog output/1(Compass Heading)

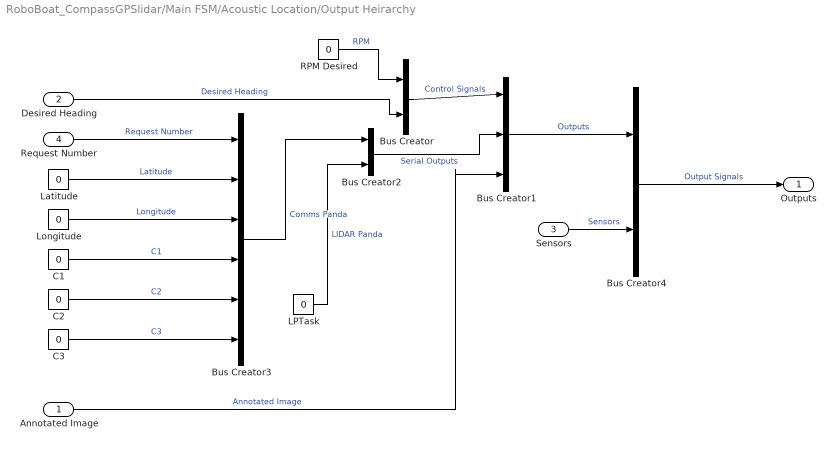
== system RoboBoat_CompassGPSlidar/Main FSM/Acoustic Location/Output Heirarchy ==
  Annotated Image : Inport
  Desired Heading : Inport  Port=2
  Sensors : Inport  Port=3
  Request Number : Inport  Port=4
  Bus Creator : BusCreator  Inputs=2
  Bus Creator1 : BusCreator  Inputs=3
  Bus Creator2 : BusCreator  Inputs=2
  Bus Creator3 : BusCreator  Inputs=6
  Bus Creator4 : BusCreator  Inputs=2
  C1 : Constant  Value=0
  C2 : Constant  Value=0
  C3 : Constant  Value=0
  LPTask : Constant  Value=0
  Latitude : Constant  Value=0
  Longitude : Constant  Value=0
  RPM Desired : Constant  Value=0
  Outputs : Outport
  wires:
  RPM Desired/1 -> Bus Creator/1  "RPM"
  Bus Creator/1 -> Bus Creator1/1  "Control Signals"
  Bus Creator3/1 -> Bus Creator2/1  "Comms Panda"
  Request Number/1 -> Bus Creator3/1  "Request Number"
  Latitude/1 -> Bus Creator3/2  "Latitude"
  Longitude/1 -> Bus Creator3/3  "Longitude"
  C1/1 -> Bus Creator3/4  "C1"
  LPTask/1 -> Bus Creator2/2  "LIDAR Panda"
  Desired Heading/1 -> Bus Creator/2  "Desired Heading"
  Bus Creator1/1 -> Bus Creator4/1  "Outputs"
  Annotated Image/1 -> Bus Creator1/3  "Annotated Image"
  Sensors/1 -> Bus Creator4/2  "Sensors"
  Bus Creator4/1 -> Outputs/1  "Output Signals"
  Bus Creator2/1 -> Bus Creator1/2  "Serial Outputs"
  C2/1 -> Bus Creator3/5  "C2"
  C3/1 -> Bus Creator3/6  "C3"

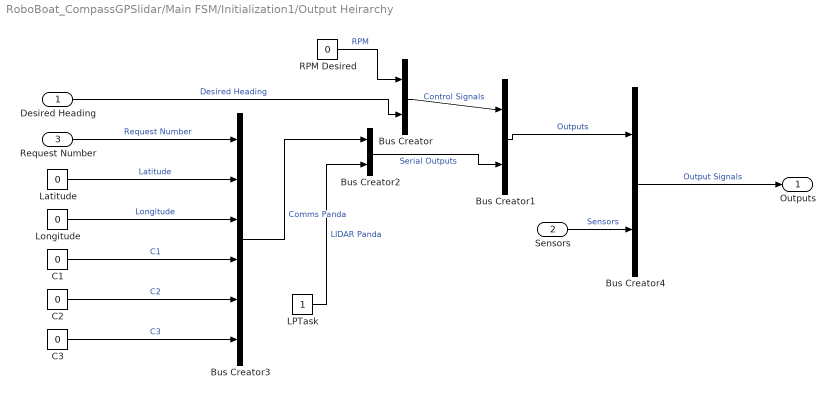
== system RoboBoat_CompassGPSlidar/Main FSM/Initialization1/Output Heirarchy ==
  Desired Heading : Inport
  Sensors : Inport  Port=2
  Request Number : Inport  Port=3
  Bus Creator{,1..2,4} (4 alike) : BusCreator  Inputs=2
  Bus Creator3 : BusCreator  Inputs=6
  C1 : Constant  Value=0
  C2 : Constant  Value=0
  C3 : Constant  Value=0
  LPTask : Constant
  Latitude : Constant  Value=0
  Longitude : Constant  Value=0
  RPM Desired : Constant  Value=0
  Outputs : Outport
  wires:
  RPM Desired/1 -> Bus Creator/1  "RPM"
  Bus Creator/1 -> Bus Creator1/1  "Control Signals"
  Bus Creator3/1 -> Bus Creator2/1  "Comms Panda"
  Request Number/1 -> Bus Creator3/1  "Request Number"
  Latitude/1 -> Bus Creator3/2  "Latitude"
  Longitude/1 -> Bus Creator3/3  "Longitude"
  C1/1 -> Bus Creator3/4  "C1"
  LPTask/1 -> Bus Creator2/2  "LIDAR Panda"
  Desired Heading/1 -> Bus Creator/2  "Desired Heading"
  Bus Creator1/1 -> Bus Creator4/1  "Outputs"
  Sensors/1 -> Bus Creator4/2  "Sensors"
  Bus Creator4/1 -> Outputs/1  "Output Signals"
  Bus Creator2/1 -> Bus Creator1/2  "Serial Outputs"
  C2/1 -> Bus Creator3/5  "C2"
  C3/1 -> Bus Creator3/6  "C3"

== system RoboBoat_CompassGPSlidar/Main FSM/NED:Waypoint/Output Heirarchy ==
  Sensors : Inport
  RPM : Inport  Port=2
  Desired Heading : Inport  Port=3
  Bus Creator{,1..2,4} (4 alike) : BusCreator  Inputs=2
  Bus Creator3 : BusCreator  Inputs=6
  C1 : Constant  Value=0  SampleTime=-1
  C2 : Constant  Value=0  SampleTime=-1
  C3 : Constant  Value=0  SampleTime=-1
  LPTask : Constant  SampleTime=-1
  Latitude : Constant  Value=0  SampleTime=-1
  Longitude : Constant  Value=0  SampleTime=-1
  Request Number : Constant  Value=0  SampleTime=-1
  Outputs : Outport
  wires:
  Bus Creator/1 -> Bus Creator1/1  "Control Signals"
  Bus Creator3/1 -> Bus Creator2/1  "Comms Panda"
  Request Number/1 -> Bus Creator3/1  "Request Number"
  Latitude/1 -> Bus Creator3/2  "Latitude"
  Longitude/1 -> Bus Creator3/3  "Longitude"
  C1/1 -> Bus Creator3/4  "C1"
  LPTask/1 -> Bus Creator2/2  "LIDAR Panda"
  Bus Creator1/1 -> Bus Creator4/1  "Outputs"
  Sensors/1 -> Bus Creator4/2  "Sensors"
  Bus Creator4/1 -> Outputs/1  "Output Signals"
  Bus Creator2/1 -> Bus Creator1/2  "Serial Outputs"
  C2/1 -> Bus Creator3/5  "C2"
  C3/1 -> Bus Creator3/6  "C3"
  RPM/1 -> Bus Creator/1  "RPM"
  Desired Heading/1 -> Bus Creator/2  "Desired Heading"

== system RoboBoat_CompassGPSlidar/Main FSM/Obstacle Navigation1/Communication ==
  Sensors : Inport
  RGB Image : Inport  Port=2
  Enable : EnablePort  ShowOutputPort=on
  Bus Selector : BusSelector  OutputSignals=Serial In.Compass.Heading
  Compare To Constant : simulink/Logic and Bit Operations/Compare To Constant  relop=>=  const=5  OutDataTypeStr=boolean
  Constant : Constant  Value=3
  Constant1 : Constant  Value=3
  Data Store Write : DataStoreWrite  DataStoreName=enterGate
  Data Store Write1 : DataStoreWrite  DataStoreName=exitGate
  Data Type Conversion : DataTypeConversion  OutDataTypeStr=double
  Discrete-Time Integrator : DiscreteIntegrator  SampleTime=0.1  ICPrevOutput=DiscIntNeverNeededParam  ICPrevScaledInput=DiscIntNeverNeededParam
  Insert Text : visiontextngfix/Insert Text  inputType=Obsolete  theText='Communication1'  getTextLocFrom=Specify via dialog  textLoc=[1 1]  getTextColorFrom=Specify via dialog  textColor=[0 0 0]  getTextIntensityFrom=Specify via dialog  textIntensity=0  getTextOpacityFrom=Specify via dialog  textOpacity=1.0  dummyVar2=0  dummyVar3=0  dummyVar4=0  imagePorts=One multidimensional signal  isInputTransposed=off  fontFace=LucidaSansRegular  dummyVar1=0  blockFontSize=12  antiAliased=on
  Output Heirarchy1 : Subsystem
  Outputs : Outport
  Finished : Outport  Port=2
  wires:
  Constant/1 -> Data Store Write/1
  Constant1/1 -> Data Store Write1/1
  Insert Text/1 -> Output Heirarchy1/3(Annotated Image)
  RGB Image/1 -> Insert Text/1
  Sensors/1 -> Bus Selector/1, Output Heirarchy1/2(Sensors)
  Bus Selector/1 -> Output Heirarchy1/1(Desired Heading)  "<Heading>"
  Enable/1 -> Discrete-Time Integrator/1
  Discrete-Time Integrator/1 -> Compare To Constant/1
  Data Type Conversion/1 -> Finished/1
  Compare To Constant/1 -> Data Type Conversion/1
  Output Heirarchy1/1(Outputs) -> Outputs/1

== system RoboBoat_CompassGPSlidar/Main FSM/Obstacle Navigation1/Enter Gate ==
  Sensors : Inport
  RGB Image : Inport  Port=2
  Enable : EnablePort
  Data Store Read : DataStoreRead  DataStoreName=enterGate
  Gate 1 (Red & White) : Subsystem  TreatAsAtomicUnit=on
  Gate 2 (White & White) : Subsystem  TreatAsAtomicUnit=on
  Gate 3 (White & Green) : Subsystem  TreatAsAtomicUnit=on
  MATLAB Function : MATLAB Function  TreatAsAtomicUnit=on
  Multiport Switch : MultiPortSwitch
  Output Reassign : Subsystem
  Outputs : Outport
  Finished : Outport  Port=2
  wires:
  Data Store Read/1 -> MATLAB Function/1(gateID)
  MATLAB Function/2(gate1En) -> Gate 1 (Red & White)/Enable
  MATLAB Function/3(gate2En) -> Gate 2 (White & White)/Enable
  MATLAB Function/4(gate3En) -> Gate 3 (White & Green)/Enable
  RGB Image/1 -> Gate 1 (Red & White)/2(RGB image), Gate 2 (White & White)/2(RGB image), Gate 3 (White & Green)/2(RGB image)
  Sensors/1 -> Gate 1 (Red & White)/1(Sensors), Gate 2 (White & White)/1(Sensors), Gate 3 (White & Green)/1(Sensors)
  Gate 1 (Red & White)/1(Outputs) -> Multiport Switch/2
  Gate 2 (White & White)/1(Outputs) -> Multiport Switch/3
  Gate 3 (White & Green)/1(Outputs) -> Multiport Switch/4
  MATLAB Function/1(outputSelector) -> Multiport Switch/1
  Multiport Switch/1 -> Output Reassign/1(Outputs in)
  Output Reassign/1(Outputs) -> Outputs/1
  Output Reassign/2(Finished) -> Finished/1

== system RoboBoat_CompassGPSlidar/Main FSM/Obstacle Navigation1/Exit Gate ==
  Sensors : Inport
  RGB Image : Inport  Port=2
  Enable : EnablePort
  Data Store Read : DataStoreRead  DataStoreName=exitGate
  Gate 1 (Red & White) : Subsystem  TreatAsAtomicUnit=on
  Gate 2 (White & White) : Subsystem  TreatAsAtomicUnit=on
  Gate 3 (White & Green) : Subsystem  TreatAsAtomicUnit=on
  MATLAB Function : MATLAB Function  TreatAsAtomicUnit=on
  Multiport Switch : MultiPortSwitch
  Outputs : Outport
  wires:
  Data Store Read/1 -> MATLAB Function/1(gateID)
  MATLAB Function/2(gate1En) -> Gate 1 (Red & White)/Enable
  MATLAB Function/3(gate2En) -> Gate 2 (White & White)/Enable
  MATLAB Function/4(gate3En) -> Gate 3 (White & Green)/Enable
  RGB Image/1 -> Gate 1 (Red & White)/2(RGB image), Gate 2 (White & White)/2(RGB image), Gate 3 (White & Green)/2(RGB image)
  Sensors/1 -> Gate 1 (Red & White)/1(Sensors), Gate 2 (White & White)/1(Sensors), Gate 3 (White & Green)/1(Sensors)
  Gate 1 (Red & White)/1(Outputs) -> Multiport Switch/2
  Gate 2 (White & White)/1(Outputs) -> Multiport Switch/3
  Gate 3 (White & Green)/1(Outputs) -> Multiport Switch/4
  MATLAB Function/1(outputSelector) -> Multiport Switch/1
  Multiport Switch/1 -> Outputs/1

== system RoboBoat_CompassGPSlidar/Main FSM/Obstacle Navigation1/GPS: Center ==
  Sensors : Inport
  RGB image : Inport  Port=2
  Enable : EnablePort
  Approach : Subsystem  TreatAsAtomicUnit=on
  GPS Enabler : MATLAB Function  TreatAsAtomicUnit=on
  GPS Selector : MultiPortSwitch  Inputs=2
  Orient : Subsystem  TreatAsAtomicUnit=on
  Output Reassign : Subsystem
  Unit Delay : UnitDelay  SampleTime=-1
  Outputs : Outport
  Finished : Outport  Port=2
  wires:
  Output Reassign/1(Outputs) -> Outputs/1
  Output Reassign/2(Finished) -> Finished/1
  Sensors/1 -> Approach/1(Sensors), Orient/1(Sensors)
  GPS Enabler/2(OrientEnable) -> Orient/Enable
  GPS Enabler/3(ApproachEnable) -> Approach/Enable
  Orient/2(Finished) -> Unit Delay/1
  Orient/1(Outputs) -> GPS Selector/2
  Approach/1(Outputs) -> GPS Selector/3
  GPS Enabler/1(GPSMode) -> GPS Selector/1
  Unit Delay/1 -> GPS Enabler/1(Finished)
  GPS Selector/1 -> Output Reassign/1(Outputs in)
  RGB image/1 -> Approach/2(RGB image), Orient/2(RGB image)

== system RoboBoat_CompassGPSlidar/Main FSM/Obstacle Navigation1/Obstacle Navigation ==
  Sensors : Inport
  RGB Image : Inport  Port=2
  Enable : EnablePort
  Data Store Read : DataStoreRead  DataStoreName=dodgeStart
  Dodge : Subsystem  TreatAsAtomicUnit=on
  GPS: Bee Line : Subsystem  TreatAsAtomicUnit=on
  MATLAB Function : MATLAB Function  TreatAsAtomicUnit=on
  Multiport Switch : MultiPortSwitch  Inputs=2
  Output Reassign : Subsystem
  Unit Delay : UnitDelay  SampleTime=-1
  Outputs : Outport
  Finished : Outport  Port=2
  wires:
  MATLAB Function/3(GPSEn) -> GPS: Bee Line/Enable
  Sensors/1 -> GPS: Bee Line/1(Sensors), Dodge/1(Sensors)
  RGB Image/1 -> GPS: Bee Line/2(RGB image), Dodge/2(RGB image)
  MATLAB Function/2(dodgeEn) -> Dodge/Enable
  Dodge/1(Outputs) -> Multiport Switch/2
  GPS: Bee Line/1(Outputs) -> Multiport Switch/3
  MATLAB Function/1(taskSelector) -> Multiport Switch/1
  Dodge/2(Dodge Incomplete) -> Unit Delay/1  "Dodge Incomplete"
  Data Store Read/1 -> MATLAB Function/2(dodgeStart)
  Unit Delay/1 -> MATLAB Function/1(dodgeIncomplete)
  Multiport Switch/1 -> Output Reassign/1(Outputs in)
  Output Reassign/1(Outputs) -> Outputs/1
  Output Reassign/2(Finished) -> Finished/1

== system RoboBoat_CompassGPSlidar/Main FSM/Obstacle Navigation1/Output Reassign ==
  Outputs in : Inport
  Bus Selector : BusSelector  OutputSignals=Task Finished,Output Signals
  Outputs : Outport
  Finished : Outport  Port=2
  wires:
  Outputs in/1 -> Bus Selector/1
  Bus Selector/1 -> Finished/1  "<Task Finished>"
  Bus Selector/2 -> Outputs/1  "<Output Signals>"

== system RoboBoat_CompassGPSlidar/Main FSM/Obstacle Navigation1/Task Option1 ==
  note: Obstacle Nav Options
  Message Composer : MATLAB Function  TreatAsAtomicUnit=on
  Obstacle Nav : Constant  Value=uint8('12345678')  SampleTime=0.1
  Option : Outport
  wires:
  Obstacle Nav/1 -> Message Composer/1(taskStrInit)
  Message Composer/1(taskStrAdj) -> Option/1

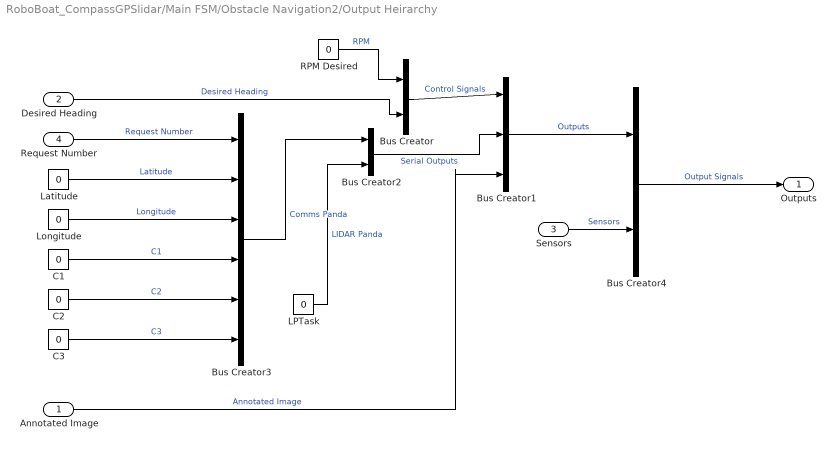
== system RoboBoat_CompassGPSlidar/Main FSM/Obstacle Navigation2/Output Heirarchy ==
  Annotated Image : Inport
  Desired Heading : Inport  Port=2
  Sensors : Inport  Port=3
  Request Number : Inport  Port=4
  Bus Creator : BusCreator  Inputs=2
  Bus Creator1 : BusCreator  Inputs=3
  Bus Creator2 : BusCreator  Inputs=2
  Bus Creator3 : BusCreator  Inputs=6
  Bus Creator4 : BusCreator  Inputs=2
  C1 : Constant  Value=0
  C2 : Constant  Value=0
  C3 : Constant  Value=0
  LPTask : Constant  Value=0
  Latitude : Constant  Value=0
  Longitude : Constant  Value=0
  RPM Desired : Constant  Value=0
  Outputs : Outport
  wires:
  RPM Desired/1 -> Bus Creator/1  "RPM"
  Bus Creator/1 -> Bus Creator1/1  "Control Signals"
  Bus Creator3/1 -> Bus Creator2/1  "Comms Panda"
  Request Number/1 -> Bus Creator3/1  "Request Number"
  Latitude/1 -> Bus Creator3/2  "Latitude"
  Longitude/1 -> Bus Creator3/3  "Longitude"
  C1/1 -> Bus Creator3/4  "C1"
  LPTask/1 -> Bus Creator2/2  "LIDAR Panda"
  Desired Heading/1 -> Bus Creator/2  "Desired Heading"
  Bus Creator1/1 -> Bus Creator4/1  "Outputs"
  Annotated Image/1 -> Bus Creator1/3  "Annotated Image"
  Sensors/1 -> Bus Creator4/2  "Sensors"
  Bus Creator4/1 -> Outputs/1  "Output Signals"
  Bus Creator2/1 -> Bus Creator1/2  "Serial Outputs"
  C2/1 -> Bus Creator3/5  "C2"
  C3/1 -> Bus Creator3/6  "C3"

== system RoboBoat_CompassGPSlidar/Main FSM/RCHold/Output Heirarchy ==
  Desired Heading : Inport
  Sensors : Inport  Port=2
  Bus Creator{,1..2,4} (4 alike) : BusCreator  Inputs=2
  Bus Creator3 : BusCreator  Inputs=6
  C1 : Constant  Value=0
  C2 : Constant  Value=0
  C3 : Constant  Value=0
  LPTask : Constant  Value=0
  Latitude : Constant  Value=0
  Longitude : Constant  Value=0
  RPM Desired : Constant  Value=0
  Request Number : Constant  Value=0
  Outputs : Outport
  wires:
  RPM Desired/1 -> Bus Creator/1  "RPM"
  Bus Creator/1 -> Bus Creator1/1  "Control Signals"
  Bus Creator3/1 -> Bus Creator2/1  "Comms Panda"
  Request Number/1 -> Bus Creator3/1  "Request Number"
  Latitude/1 -> Bus Creator3/2  "Latitude"
  Longitude/1 -> Bus Creator3/3  "Longitude"
  C1/1 -> Bus Creator3/4  "C1"
  LPTask/1 -> Bus Creator2/2  "LIDAR Panda"
  Desired Heading/1 -> Bus Creator/2  "Desired Heading"
  Bus Creator1/1 -> Bus Creator4/1  "Outputs"
  Sensors/1 -> Bus Creator4/2  "Sensors"
  Bus Creator4/1 -> Outputs/1  "Output Signals"
  Bus Creator2/1 -> Bus Creator1/2  "Serial Outputs"
  C2/1 -> Bus Creator3/5  "C2"
  C3/1 -> Bus Creator3/6  "C3"
